simulink model "prblm6"  (R2020b)
settings: Solver=VariableStepAuto  StartTime=0.0  StopTime=10.0  RelTol=1e-3
settings Model: Creator=shridhar  LastModifiedBy=shridhar

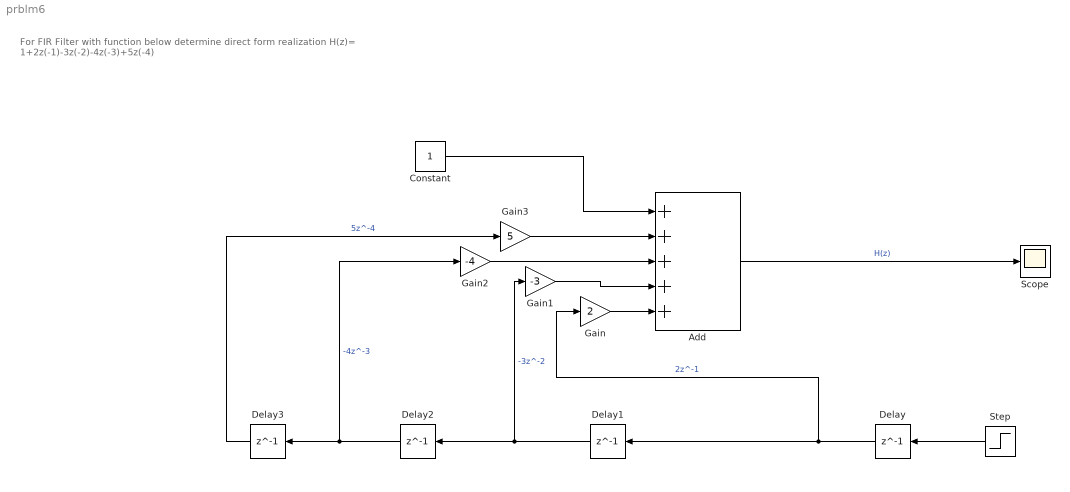
== system prblm6 ==
  note: For FIR Filter with function below determine direct form realization
      | H(z)= 1+2z(-1)-3z(-2)-4z(-3)+5z(-4)
  Add : Sum  Inputs=+++++
  Constant : Constant
  Delay{,1..3} (4 alike) : Delay  DelayLength=1
  Gain : Gain  Gain=2
  Gain1 : Gain  Gain=-3
  Gain2 : Gain  Gain=-4
  Gain3 : Gain  Gain=5
  Scope : Scope
  Step : Step  SampleTime=0
  wires:
  Add/1 -> Scope/1  "H(z)"
  Delay2/1 -> Gain2/1, Delay3/1  "-4z^-3"
  Delay1/1 -> Gain1/1, Delay2/1  "-3z^-2"
  Delay/1 -> Gain/1, Delay1/1  "2z^-1"
  Step/1 -> Delay/1
  Constant/1 -> Add/1
  Gain/1 -> Add/5
  Gain1/1 -> Add/4
  Gain2/1 -> Add/3
  Delay3/1 -> Gain3/1  "5z^-4"
  Gain3/1 -> Add/2
